simulink model "flightControlSystem"  (R2019a)
settings: Solver=ode3  StartTime=0  StopTime=TFinal  FixedStep=Ts  RelTol=1e-3  EnableMultiTasking=on
undefined symbols (not defined in the file): codertarget, controlModePosVSOrient, enableLanding, Estimator, landCommand, landingAltitude, live_time_ticks, orient_ref, pos_ref, Rec, SDTV, takeoff_flag, takeoffCommand, takeOffDuration, TFinal, Ts, x_target, y_target, z_target
libraries: simulink x5, parrotlib x3, SignalEditorBlockLib x1, sharedtransform x1, visionstatistics x1, visionconversions x1
settings Model: ExtModeTrigDuration=80  Creator=The MathWorks, Inc.  LastModifiedBy=umwan492
settings DataIOCC: LimitDataPoints=on  SaveFormat=StructureWithTime  ReturnWorkspaceOutputs=off
settings OptimizationCC: BlockReduction=off  EnhancedBackFolding=on  PassReuseOutputArgsAs=Individual arguments  MaxStackSize=64  OptimizeBlockOrder=speed  DifferentSizesBufferReuse=on  OptimizationCustomize=off
settings DebuggingCC: AlgebraicLoopMsg=none  IntegerOverflowMsg=none  ParameterPrecisionLossMsg=none  ParameterTunabilityLossMsg=error  UnconnectedInputMsg=none  UnconnectedOutputMsg=none  UnconnectedLineMsg=none  BusObjectLabelMismatch=error  PregeneratedLibrarySubsystemCodeDiagnostic=none  SFUnexpectedBacktrackingDiag=warning  SFNoUnconditionalDefaultTransitionDiag=warning  SFExecutionAtInitializationDiag=none  IntegerSaturationMsg=none  ArithmeticOperatorsInVariantConditions=warning
settings HardwareCC: ProdBitPerPointer=32  ProdBitPerSizeT=32  ProdBitPerPtrDiffT=32  ProdLargestAtomicInteger=Long  ProdWordSize=32  ProdHWDeviceType=ARM Compatible->ARM 9
settings ModelReferenceCC: ModelReferenceNumInstancesAllowed=Single  PropagateSignalLabelsOutOfModel=off
settings SFSimCC: SimUseLocalCustomCode=off  MATLABDynamicMemAlloc=off
settings RTWCC: SystemTargetFile=ert.tlc  HardwareBoard=PARROT Mambo  TLCOptions=-aInlineSetEventsForThisBaseRateFcn=TLC_FALSE -aSuppressMultiTaskScheduler=TLC_FALSE -aRateBasedStepFcn=1  TemplateMakefile=ert_default_tmf  GenerateReport=on  RTWUseLocalCustomCode=off  Toolchain=Sourcery G++ Lite GNU Toolchain for Drones  IncludeHyperlinkInReport=on  LaunchReport=on  GenerateTraceInfo=on  GenerateTraceReport=on  GenerateTraceReportSl=on  GenerateTraceReportSf=on  GenerateTraceReportEml=on
settings CodeAppCC: ForceParamTrailComments=on  IgnoreCustomStorageClasses=off  MaxIdLength=63  OperatorAnnotations=on  SimulinkDataObjDesc=on  SFDataObjDesc=on  InsertBlockDesc=on
settings ERTTargetCC: MatFileLogging=on  SupportContinuousTime=on
settings ConfigComp: CovMetricSettings=dw  CovHtmlReporting=on  CovSaveCumulativeToWorkspaceVar=on  CovSaveSingleToWorkspaceVar=on  CovExternalEMLEnable=off  CovSFcnEnable=off

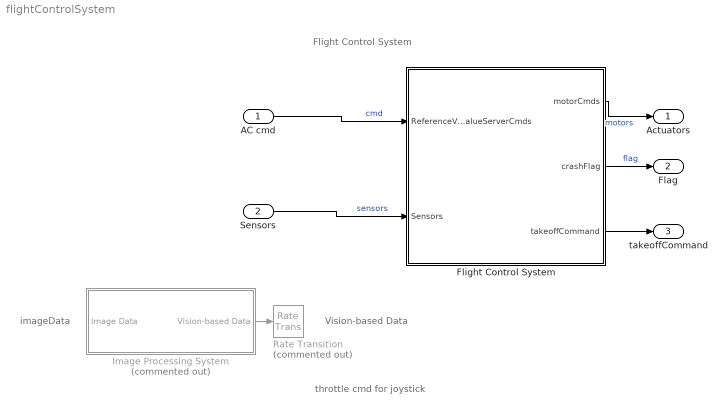
== system flightControlSystem ==
  note: throttle cmd for joystick
  note: Vision-based Data
  note: imageData
  note: Flight Control System
  AC cmd : Inport  OutDataTypeStr=Bus: CommandBus  BusOutputAsStruct=on
  Sensors : Inport  Port=2  OutDataTypeStr=Bus: SensorsBus  BusOutputAsStruct=on
  Flight Control System : Subsystem  TreatAsAtomicUnit=on
  Image Processing System : Subsystem  Tag=IP_SUB  Commented=on  InitFcn=codertarget.parrot.internal.ipSubsystemCallback(gcb);  TreatAsAtomicUnit=on  SystemSampleTime=40*Ts  RTWFcnName=ImageFunction
      settings: RTWSystemCode=Inline  RTWFcnNameOpts=User specified
  Rate Transition : RateTransition  Commented=on  Deterministic=off
  Actuators : Outport  OutDataTypeStr=single  PortDimensions=4
  Flag : Outport  Port=2  OutDataTypeStr=uint8  PortDimensions=1
  takeoffCommand : Outport  Port=3  OutDataTypeStr=boolean  PortDimensions=1
  wires:
  AC cmd/1 -> Flight Control System/1(ReferenceValueServerCmds)  "cmd"
  Flight Control System/1(motorCmds) -> Actuators/1  "motors"
  Sensors/1 -> Flight Control System/2(Sensors)  "sensors"
  Flight Control System/2(crashFlag) -> Flag/1  "flag"
  Image Processing System/1(Vision-based Data) -> Rate Transition/1
  Flight Control System/3(takeoffCommand) -> takeoffCommand/1

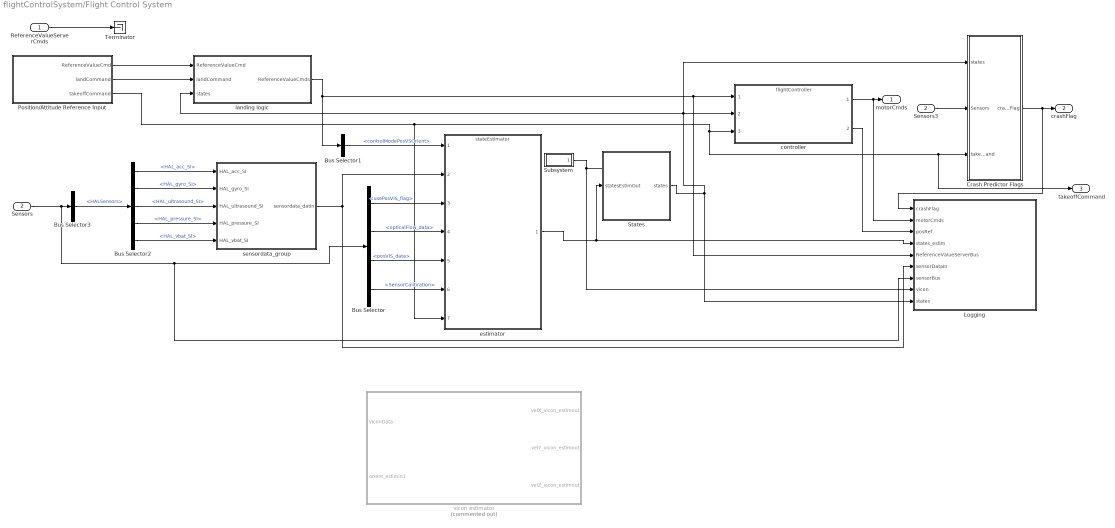
== system flightControlSystem/Flight Control System ==
  ReferenceValueServerCmds : Inport  OutDataTypeStr=Bus: CommandBus
  Sensors : Inport  Port=2  OutDataTypeStr=Bus: SensorsBus  BusOutputAsStruct=on
  Bus Selector : BusSelector  OutputSignals=VisionSensors.usePosVIS_flag,VisionSensors.opticalFlow_data,VisionSensors.posVIS_data,SensorCalibration
  Bus Selector1 : BusSelector  OutputSignals=controlModePosVSOrient
  Bus Selector2 : BusSelector  OutputSignals=HAL_acc_SI,HAL_gyro_SI,HAL_ultrasound_SI,HAL_pressure_SI,HAL_vbat_SI
  Bus Selector3 : BusSelector  OutputSignals=HALSensors
  Crash Predictor Flags : Subsystem
  Logging : Subsystem  TreatAsAtomicUnit=on
      settings: RTWFcnNameOpts=Use subsystem name
  Position/Attitude Reference Input : Subsystem
  Sensors3 : InportShadow  Port=2  OutDataTypeStr=Bus: SensorsBus  BusOutputAsStruct=on
  States : Subsystem
  Subsystem : Subsystem
  Terminator : Terminator
  controller : ModelReference  ModelNameDialog=flightController.slx  SimulationMode=Normal  ModelReferenceVersion=1.190
  estimator : ModelReference  ModelNameDialog=stateEstimator.slx  SimulationMode=Normal  ModelReferenceVersion=1.78
  landing logic : Subsystem
  sensordata_group : Subsystem
  vicon estimator : Subsystem  Commented=on
  motorCmds : Outport
  crashFlag : Outport  Port=2
  takeoffCommand : Outport  Port=3  OutDataTypeStr=boolean
  wires:
  Bus Selector2/1 -> sensordata_group/1(HAL_acc_SI)  "<HAL_acc_SI>"
  Bus Selector2/2 -> sensordata_group/2(HAL_gyro_SI)  "<HAL_gyro_SI>"
  Bus Selector2/4 -> sensordata_group/4(HAL_pressure_SI)  "<HAL_pressure_SI>"
  Bus Selector2/3 -> sensordata_group/3(HAL_ultrasound_SI)  "<HAL_ultrasound_SI>"
  estimator/1 -> States/1(statesEstimOut), Logging/4(states_estim)
  controller/2 -> Logging/3(posRef)
  landing logic/1(ReferenceValueCmds) -> Logging/5(ReferenceValueServerBus), controller/1, Bus Selector1/1
  controller/1 -> motorCmds/1, Logging/2(motorCmds)
  sensordata_group/1(sensordata_datin) -> Logging/6(sensorDataIn), estimator/2
  Bus Selector2/5 -> sensordata_group/5(HAL_vbat_SI)  "<HAL_vbat_SI>"
  Crash Predictor Flags/1(crashFlag) -> Logging/1(crashFlag), crashFlag/1
  Sensors/1 -> Logging/7(sensorBus), Bus Selector/1, Bus Selector3/1
  Bus Selector3/1 -> Bus Selector2/1  "<HALSensors>"
  Bus Selector/1 -> estimator/3  "<usePosVIS_flag>"
  Bus Selector/2 -> estimator/4  "<opticalFlow_data>"
  Bus Selector/3 -> estimator/5  "<posVIS_data>"
  Bus Selector/4 -> estimator/6  "<SensorCalibration>"
  Bus Selector1/1 -> estimator/1  "<controlModePosVSOrient>"
  ReferenceValueServerCmds/1 -> Terminator/1
  Position/Attitude Reference Input/1(ReferenceValueCmd) -> landing logic/1(ReferenceValueCmd)
  Sensors3/1 -> Crash Predictor Flags/2(Sensors)
  States/1(states) -> controller/2, landing logic/3(states), Crash Predictor Flags/1(states), Logging/9(states)
  Subsystem/1(viconData) -> Logging/8(vicon)
  Position/Attitude Reference Input/2(landCommand) -> landing logic/2(landCommand)
  Position/Attitude Reference Input/3(takeoffCommand) -> estimator/7, controller/3, takeoffCommand/1, Crash Predictor Flags/3(takeoffCommand)

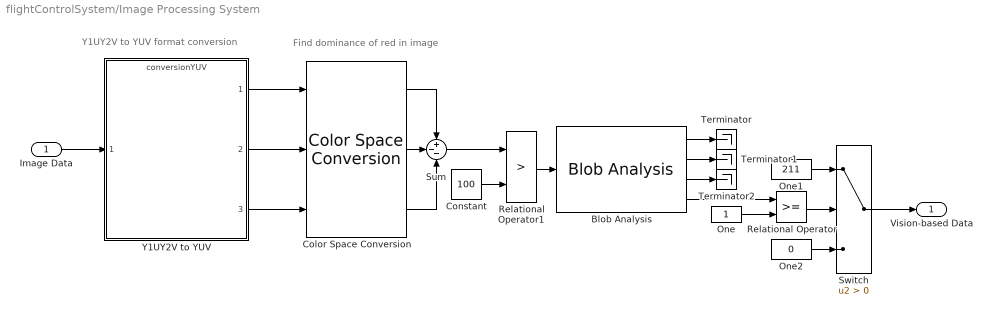
== system flightControlSystem/Image Processing System ==
  note: Find dominance of red in image
  note: Y1UY2V to YUV format conversion
  Image Data : Inport
  Blob Analysis : visionstatistics/Blob Analysis  Tag=vipblks_row_conv  area=on  centroid=on  bBox=on  majorAxis=off  minorAxis=off  angle=off  eccentricity=off  equivDiameterSq=off  extent=off  perimeter=off  outDT=single  conn=8  isLabel=off  maxBlobs=50  warnIfNumBlobsExceeded=on  isCount=on  useMinArea=off  minArea=0  useMaxArea=off  maxArea=intmax('uint32')  excludeBorderBlob=off  isOutVarDim=off  isFill=on  fillValues=-1  roundingMode=Floor  overflowMode=off  prodOutputMode=Binary point scaling  prodOutputWordLength=32  prodOutputFracLength=16  prodOutputSlope=2^-16  accumMode=Binary point scaling  accumWordLength=32  accumFracLength=0  accumSlope=2^0  outputMode=Binary point scaling  outputWordLength=32  outputFracLength=16  outputSlope=2^-16  memorySlope=2^-16  firstCoeffMode=Binary point scaling  firstCoeffWordLength=16  firstCoeffFracLength=14  firstCoeffSlope=2^-14  secondCoeffMode=Binary point scaling  secondCoeffWordLength=32  secondCoeffFracLength=16  secondCoeffSlope=2^-16
      settings: SourceProductName=Computer Vision Toolbox
  Color Space Conversion : visionconversions/Color Space  Conversion  conversion=Obsolete  conversionActive=Y'CbCr to R'G'B'  wp_str=D65  rec=Rec. 601 (SDTV)  sys=1125/60/2:1  imagePorts=Separate color signals
  Constant : Constant  Value=100  OutDataTypeStr=uint8
  One : Constant  OutDataTypeStr=Inherit: Inherit via back propagation
  One1 : Constant  Value=211  OutDataTypeStr=Inherit: Inherit via back propagation
  One2 : Constant  Value=0  OutDataTypeStr=Inherit: Inherit via back propagation
  Relational Operator : RelationalOperator  OutDataTypeStr=boolean  RndMeth=Simplest
  Relational Operator1 : RelationalOperator  Operator=>  OutDataTypeStr=boolean  RndMeth=Simplest
  Sum : Sum  Inputs=+--  SaturateOnIntegerOverflow=on
  Switch : Switch  Criteria=u2 > Threshold
  Terminator : Terminator
  Terminator1 : Terminator
  Terminator2 : Terminator
  Y1UY2V to YUV : ModelReference  ModelNameDialog=conversionYUV.slx  SimulationMode=Normal  ModelReferenceVersion=1.145
  Vision-based Data : Outport
  wires:
  One/1 -> Relational Operator/2
  Blob Analysis/4 -> Relational Operator/1
  Relational Operator1/1 -> Blob Analysis/1
  Color Space Conversion/1 -> Sum/1
  Color Space Conversion/2 -> Sum/2
  Color Space Conversion/3 -> Sum/3
  Sum/1 -> Relational Operator1/1
  Constant/1 -> Relational Operator1/2
  Blob Analysis/1 -> Terminator/1
  Blob Analysis/2 -> Terminator1/1
  Blob Analysis/3 -> Terminator2/1
  Relational Operator/1 -> Switch/2
  Switch/1 -> Vision-based Data/1
  One1/1 -> Switch/1
  One2/1 -> Switch/3
  Image Data/1 -> Y1UY2V to YUV/1
  Y1UY2V to YUV/1 -> Color Space Conversion/1
  Y1UY2V to YUV/2 -> Color Space Conversion/2
  Y1UY2V to YUV/3 -> Color Space Conversion/3

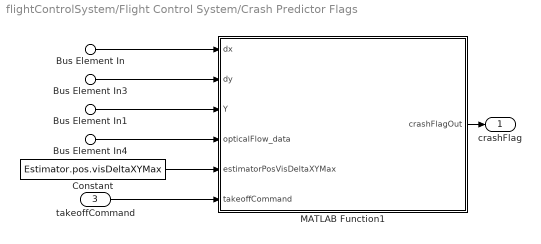
== system flightControlSystem/Flight Control System/Crash Predictor Flags ==
  Bus Element In1 : Inport  PortName=states  Element=Y
  Bus Element In : Inport  PortName=states  Element=dx
  Bus Element In3 : Inport  PortName=states  Element=dy
  Bus Element In4 : Inport  Port=2  PortName=Sensors  Element=VisionSensors.opticalFlow_data
  takeoffCommand : Inport  Port=3
  Constant : Constant  Value=Estimator.pos.visDeltaXYMax
  MATLAB Function1 : MATLAB Function  TreatAsAtomicUnit=on
  crashFlag : Outport
  wires:
  Bus Element In4/1 -> MATLAB Function1/4(opticalFlow_data)
  MATLAB Function1/1(crashFlagOut) -> crashFlag/1
  Bus Element In3/1 -> MATLAB Function1/2(dy)
  Constant/1 -> MATLAB Function1/5(estimatorPosVisDeltaXYMax)
  Bus Element In/1 -> MATLAB Function1/1(dx)
  takeoffCommand/1 -> MATLAB Function1/6(takeoffCommand)
  Bus Element In1/1 -> MATLAB Function1/3(Y)

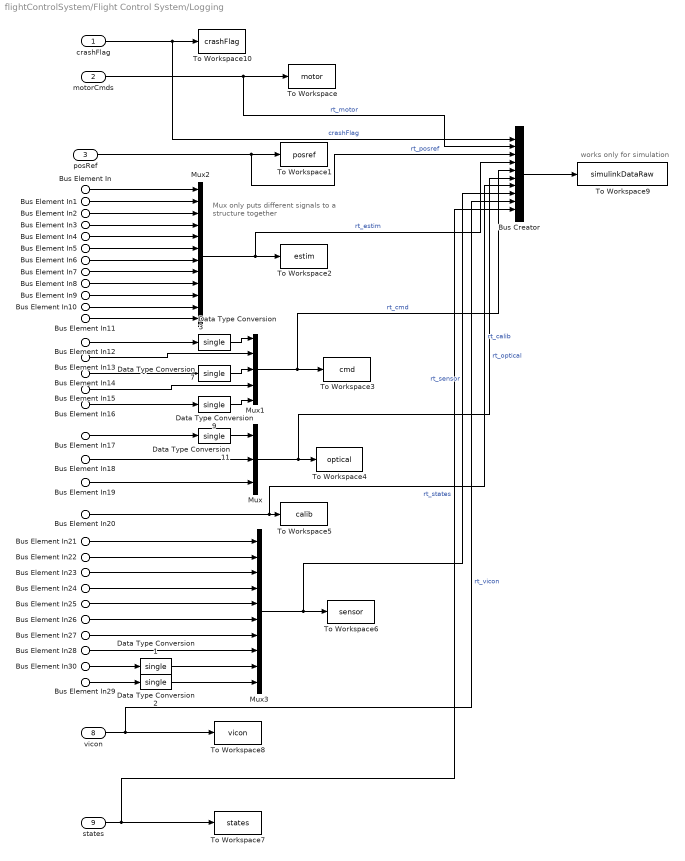
== system flightControlSystem/Flight Control System/Logging ==
  note: works only for simulation
  note: Mux only puts different signals to a structure together
  crashFlag : Inport
  motorCmds : Inport  Port=2
  posRef : Inport  Port=3
  Bus Element In : Inport  Port=4  PortName=states_estim  Element=X
  Bus Element In1 : Inport  Port=4  PortName=states_estim  Element=Y
  Bus Element In2 : Inport  Port=4  PortName=states_estim  Element=Z
  Bus Element In3 : Inport  Port=4  PortName=states_estim  Element=yaw
  Bus Element In6 : Inport  Port=4  PortName=states_estim  Element=dx
  Bus Element In5 : Inport  Port=4  PortName=states_estim  Element=roll
  Bus Element In4 : Inport  Port=4  PortName=states_estim  Element=pitch
  Bus Element In7 : Inport  Port=4  PortName=states_estim  Element=dy
  Bus Element In8 : Inport  Port=4  PortName=states_estim  Element=dz
  Bus Element In9 : Inport  Port=4  PortName=states_estim  Element=p
  Bus Element In10 : Inport  Port=4  PortName=states_estim  Element=q
  Bus Element In11 : Inport  Port=4  PortName=states_estim  Element=r
  Bus Element In12 : Inport  Port=5  PortName=ReferenceValueServerBus  Element=controlModePosVSOrient
  Bus Element In13 : Inport  Port=5  PortName=ReferenceValueServerBus  Element=pos_ref
  Bus Element In14 : Inport  Port=5  PortName=ReferenceValueServerBus  Element=takeoff_flag
  Bus Element In15 : Inport  Port=5  PortName=ReferenceValueServerBus  Element=orient_ref
  Bus Element In16 : Inport  Port=5  PortName=ReferenceValueServerBus  Element=live_time_ticks
  Bus Element In21 : Inport  Port=6  PortName=sensorDataIn  Element=ddx
  Bus Element In22 : Inport  Port=6  PortName=sensorDataIn  Element=ddy
  Bus Element In23 : Inport  Port=6  PortName=sensorDataIn  Element=ddz
  Bus Element In24 : Inport  Port=6  PortName=sensorDataIn  Element=p
  Bus Element In25 : Inport  Port=6  PortName=sensorDataIn  Element=q
  Bus Element In26 : Inport  Port=6  PortName=sensorDataIn  Element=r
  Bus Element In27 : Inport  Port=6  PortName=sensorDataIn  Element=altitude_sonar
  Bus Element In28 : Inport  Port=6  PortName=sensorDataIn  Element=prs
  Bus Element In29 : Inport  Port=6  PortName=sensorDataIn  Element=vbat_percentage
  Bus Element In30 : Inport  Port=6  PortName=sensorDataIn  Element=vbat_V
  Bus Element In17 : Inport  Port=7  PortName=sensorBus  Element=VisionSensors.usePosVIS_flag
  Bus Element In18 : Inport  Port=7  PortName=sensorBus  Element=VisionSensors.opticalFlow_data
  Bus Element In19 : Inport  Port=7  PortName=sensorBus  Element=VisionSensors.posVIS_data
  Bus Element In20 : Inport  Port=7  PortName=sensorBus  Element=SensorCalibration
  vicon : Inport  Port=8  OutDataTypeStr=Bus: viconData
  states : Inport  Port=9  OutDataTypeStr=Bus: statesBB
  Bus Creator : BusCreator  Inputs=10
  Data Type Conversion{1..3,7,9,11} (6 alike) : DataTypeConversion  OutDataTypeStr=single
  Mux : Mux  Inputs=3
  Mux1 : Mux  Inputs=5
  Mux2 : Mux  Inputs=12
  Mux3 : Mux  Inputs=10
  To Workspace : ToWorkspace  VariableName=motor  SaveFormat=Structure With Time  SampleTime=-1
  To Workspace1 : ToWorkspace  VariableName=posref  SaveFormat=Structure With Time  SampleTime=-1
  To Workspace10 : ToWorkspace  VariableName=crashFlag  SaveFormat=Structure With Time  SampleTime=-1
  To Workspace2 : ToWorkspace  VariableName=estim  SaveFormat=Structure With Time  SampleTime=-1
  To Workspace3 : ToWorkspace  VariableName=cmd  SaveFormat=Structure With Time  SampleTime=-1
  To Workspace4 : ToWorkspace  VariableName=optical  SaveFormat=Structure With Time  SampleTime=-1
  To Workspace5 : ToWorkspace  VariableName=calib  SaveFormat=Structure With Time  SampleTime=-1
      settings: Decimation=100
  To Workspace6 : ToWorkspace  VariableName=sensor  SaveFormat=Structure With Time  SampleTime=-1
  To Workspace7 : ToWorkspace  VariableName=states  SaveFormat=Structure With Time  SampleTime=-1
  To Workspace8 : ToWorkspace  VariableName=vicon  SaveFormat=Structure With Time  SampleTime=-1
  To Workspace9 : ToWorkspace  VariableName=simulinkDataRaw  SaveFormat=Timeseries  SampleTime=-1
  wires:
  Bus Element In12/1 -> Data Type Conversion3/1
  Bus Element In14/1 -> Data Type Conversion7/1
  Bus Element In16/1 -> Data Type Conversion9/1
  Bus Element In17/1 -> Data Type Conversion11/1
  Bus Element In20/1 -> Bus Creator/7, To Workspace5/1  "rt_calib"
  Mux/1 -> Bus Creator/6, To Workspace4/1  "rt_optical"
  Mux2/1 -> Bus Creator/4, To Workspace2/1  "rt_estim"
  motorCmds/1 -> Bus Creator/2, To Workspace/1  "rt_motor"
  Mux1/1 -> Bus Creator/5, To Workspace3/1  "rt_cmd"
  Bus Element In3/1 -> Mux2/4
  Bus Element In5/1 -> Mux2/6
  Bus Element In4/1 -> Mux2/5
  Bus Element In8/1 -> Mux2/9
  Bus Element In6/1 -> Mux2/7
  Bus Element In7/1 -> Mux2/8
  Bus Element In9/1 -> Mux2/10
  Bus Element In11/1 -> Mux2/12
  Bus Element In1/1 -> Mux2/2
  Bus Element In10/1 -> Mux2/11
  Bus Element In2/1 -> Mux2/3
  Bus Element In/1 -> Mux2/1
  Data Type Conversion3/1 -> Mux1/1
  Bus Element In13/1 -> Mux1/2
  Data Type Conversion7/1 -> Mux1/3
  Bus Element In15/1 -> Mux1/4
  Data Type Conversion9/1 -> Mux1/5
  Bus Element In19/1 -> Mux/3
  Bus Element In18/1 -> Mux/2
  Data Type Conversion11/1 -> Mux/1
  posRef/1 -> Bus Creator/3, To Workspace1/1  "rt_posref"
  Bus Element In21/1 -> Mux3/1
  Bus Element In22/1 -> Mux3/2
  Bus Element In23/1 -> Mux3/3
  Bus Element In24/1 -> Mux3/4
  Bus Element In25/1 -> Mux3/5
  Bus Element In26/1 -> Mux3/6
  Bus Element In27/1 -> Mux3/7
  Bus Element In28/1 -> Mux3/8
  Bus Element In30/1 -> Data Type Conversion1/1
  Bus Element In29/1 -> Data Type Conversion2/1
  Mux3/1 -> Bus Creator/8, To Workspace6/1  "rt_sensor"
  Data Type Conversion1/1 -> Mux3/9
  Data Type Conversion2/1 -> Mux3/10
  states/1 -> Bus Creator/10, To Workspace7/1  "rt_states"
  vicon/1 -> Bus Creator/9, To Workspace8/1  "rt_vicon"
  Bus Creator/1 -> To Workspace9/1
  crashFlag/1 -> Bus Creator/1, To Workspace10/1  "crashFlag"

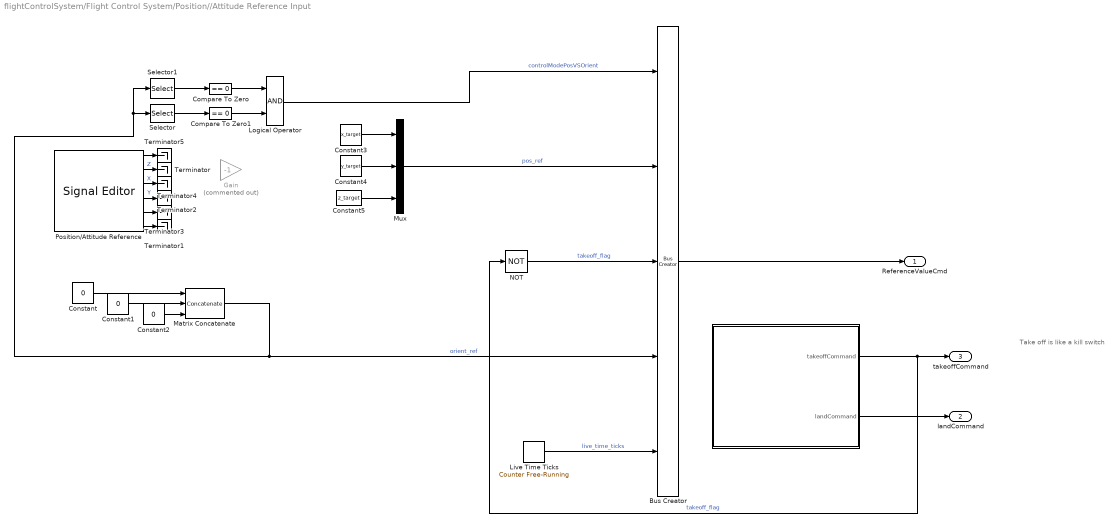
== system flightControlSystem/Flight Control System/Position//Attitude Reference Input ==
  note: Take off is like a kill switch
  " " : Subsystem  Variant=on  VariantControl=Variant1
  Bus Creator : BusCreator  Inputs=controlModePosVSOrient,pos_ref,takeoff_flag,orient_ref,live_time_ticks  OutDataTypeStr=Bus: CommandBus  NonVirtualBus=on
  Compare To Zero : simulink/Logic and Bit Operations/Compare To Zero  relop===  OutDataTypeStr=boolean
  Compare To Zero1 : simulink/Logic and Bit Operations/Compare To Zero  relop===  OutDataTypeStr=boolean
  Constant : Constant  Value=0  OutDataTypeStr=single  SampleTime=Ts
  Constant1 : Constant  Value=0  OutDataTypeStr=single  SampleTime=Ts
  Constant2 : Constant  Value=0  OutDataTypeStr=single  SampleTime=Ts
  Constant3 : Constant  Value=x_target  OutDataTypeStr=single  SampleTime=Ts
  Constant4 : Constant  Value=y_target  OutDataTypeStr=single  SampleTime=Ts
  Constant5 : Constant  Value=z_target  OutDataTypeStr=single  SampleTime=Ts
  Gain : Gain  Commented=on  Gain=-1
  Live Time Ticks : simulink/Sources/Counter Free-Running  NumBits=32  tsamp=Ts
  Logical Operator : Logic  AllPortsSameDT=off  OutDataTypeStr=boolean
  Matrix Concatenate : Concatenate  NumInputs=3  Mode=Multidimensional array  ConcatenateDimension=2
  Mux : Mux  Inputs=3
  NOT : Logic  Operator=NOT  IconShape=distinctive  AllPortsSameDT=off  OutDataTypeStr=boolean
  Position/Attitude Reference : SignalEditorBlockLib/Signal Editor  FileName=positionAttitudeRef.mat  ActiveScenario=Amin_Hover  ActiveSignal=Signal  IsBus=off  OutputBusObjectStr=Bus: BusObject  SampleTime=Ts  ZeroCross=off  OutputAfterFinalValue=Setting to zero  Unit=inherit  PreserveSignalName=on
      settings: SourceProductName=Simulink
  Selector : Selector  InputPortWidth=3  IndexOptions=Index vector (dialog)  Indices=2  OutputSizes=1
  Selector1 : Selector  InputPortWidth=3  IndexOptions=Index vector (dialog)  Indices=3  OutputSizes=1
  Terminator{,1..5} (6 alike) : Terminator
  ReferenceValueCmd : Outport
  landCommand : Outport  Port=2
  takeoffCommand : Outport  Port=3
  wires:
  Logical Operator/1 -> Bus Creator/1  "controlModePosVSOrient"
  Selector/1 -> Compare To Zero1/1
  Live Time Ticks/1 -> Bus Creator/5  "live_time_ticks"
  Compare To Zero1/1 -> Logical Operator/2
  Selector1/1 -> Compare To Zero/1
  Compare To Zero/1 -> Logical Operator/1
  Matrix Concatenate/1 -> Selector1/1, Selector/1, Bus Creator/4  "orient_ref"
  Constant/1 -> Matrix Concatenate/1
  Constant1/1 -> Matrix Concatenate/2
  Constant2/1 -> Matrix Concatenate/3
  Constant3/1 -> Mux/1
  Constant4/1 -> Mux/2
  Position/Attitude Reference/2 -> Terminator/1  "Z"
  Position/Attitude Reference/4 -> Terminator2/1  "Y"
  Position/Attitude Reference/5 -> Terminator3/1
  Position/Attitude Reference/6 -> Terminator1/1
  Position/Attitude Reference/3 -> Terminator4/1  "X"
  Position/Attitude Reference/1 -> Terminator5/1
  Constant5/1 -> Mux/3
  Mux/1 -> Bus Creator/2  "pos_ref"
  Bus Creator/1 -> ReferenceValueCmd/1
  " "/1(takeoffCommand) -> NOT/1, takeoffCommand/1  "takeoff_flag"
  " "/2(landCommand) -> landCommand/1
  NOT/1 -> Bus Creator/3  "takeoff_flag"

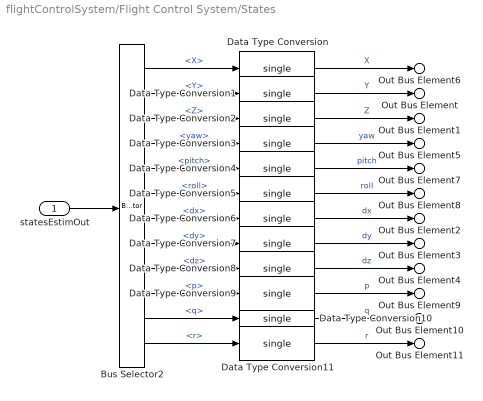
== system flightControlSystem/Flight Control System/States ==
  statesEstimOut : Inport  OutDataTypeStr=Bus: statesEstim_t
  Bus Selector2 : BusSelector  OutputSignals=X,Y,Z,yaw,pitch,roll,dx,dy,dz,p,q,r
  Data Type Conversion{,1..11} (12 alike) : DataTypeConversion  OutDataTypeStr=single
  Out Bus Element6 : Outport  PortName=states  Element=X
  Out Bus Element : Outport  PortName=states  Element=Y
  Out Bus Element1 : Outport  PortName=states  Element=Z
  Out Bus Element5 : Outport  PortName=states  Element=yaw
  Out Bus Element7 : Outport  PortName=states  Element=pitch
  Out Bus Element8 : Outport  PortName=states  Element=roll
  Out Bus Element2 : Outport  PortName=states  Element=dx
  Out Bus Element3 : Outport  PortName=states  Element=dy
  Out Bus Element4 : Outport  PortName=states  Element=dz
  Out Bus Element9 : Outport  PortName=states  Element=p
  Out Bus Element10 : Outport  PortName=states  Element=q
  Out Bus Element11 : Outport  PortName=states  Element=r
  wires:
  statesEstimOut/1 -> Bus Selector2/1
  Bus Selector2/1 -> Data Type Conversion/1  "<X>"
  Bus Selector2/2 -> Data Type Conversion1/1  "<Y>"
  Bus Selector2/3 -> Data Type Conversion2/1  "<Z>"
  Bus Selector2/4 -> Data Type Conversion3/1  "<yaw>"
  Bus Selector2/5 -> Data Type Conversion4/1  "<pitch>"
  Bus Selector2/6 -> Data Type Conversion5/1  "<roll>"
  Bus Selector2/7 -> Data Type Conversion6/1  "<dx>"
  Bus Selector2/8 -> Data Type Conversion7/1  "<dy>"
  Bus Selector2/9 -> Data Type Conversion8/1  "<dz>"
  Bus Selector2/10 -> Data Type Conversion9/1  "<p>"
  Bus Selector2/11 -> Data Type Conversion10/1  "<q>"
  Bus Selector2/12 -> Data Type Conversion11/1  "<r>"
  Data Type Conversion/1 -> Out Bus Element6/1  "X"
  Data Type Conversion1/1 -> Out Bus Element/1  "Y"
  Data Type Conversion2/1 -> Out Bus Element1/1  "Z"
  Data Type Conversion3/1 -> Out Bus Element5/1  "yaw"
  Data Type Conversion4/1 -> Out Bus Element7/1  "pitch"
  Data Type Conversion5/1 -> Out Bus Element8/1  "roll"
  Data Type Conversion6/1 -> Out Bus Element2/1  "dx"
  Data Type Conversion7/1 -> Out Bus Element3/1  "dy"
  Data Type Conversion8/1 -> Out Bus Element4/1  "dz"
  Data Type Conversion9/1 -> Out Bus Element9/1  "p"
  Data Type Conversion10/1 -> Out Bus Element10/1  "q"
  Data Type Conversion11/1 -> Out Bus Element11/1  "r"

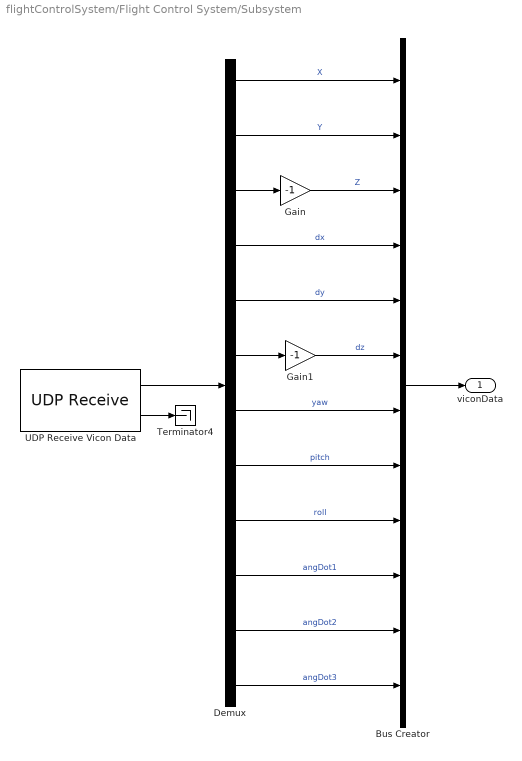
== system flightControlSystem/Flight Control System/Subsystem ==
  Bus Creator : BusCreator  Inputs=12  OutDataTypeStr=Bus: viconData
      settings: InheritFromInputs=off
  Demux : Demux  Outputs=12
  Gain : Gain  Gain=-1
  Gain1 : Gain  Gain=-1
  Terminator4 : Terminator
  UDP Receive Vicon Data : parrotlib/UDP Receive  localURL='0.0.0.0'  localPort=25000  remoteURL='0.0.0.0'  remotePort=-1  recvBufferSize=8192  signalDatatype=single  dims=12  isVarSize=off  showBlockingTime=off  blockingTime=0  sampletime=0.005  blockPlatform=LINUX
      settings: SourceProductName=Simulink Support Package for PARROT Minidrones  SourceProductBaseCode=MINIDRONES
  viconData : Outport  OutDataTypeStr=Bus: viconData
  wires:
  Demux/7 -> Bus Creator/7  "yaw"
  Demux/1 -> Bus Creator/1  "X"
  Gain/1 -> Bus Creator/3  "Z"
  Demux/10 -> Bus Creator/10  "angDot1"
  UDP Receive Vicon Data/2 -> Terminator4/1
  Demux/12 -> Bus Creator/12  "angDot3"
  Demux/5 -> Bus Creator/5  "dy"
  UDP Receive Vicon Data/1 -> Demux/1
  Demux/11 -> Bus Creator/11  "angDot2"
  Demux/2 -> Bus Creator/2  "Y"
  Gain1/1 -> Bus Creator/6  "dz"
  Demux/4 -> Bus Creator/4  "dx"
  Demux/9 -> Bus Creator/9  "roll"
  Demux/6 -> Gain1/1
  Demux/3 -> Gain/1
  Demux/8 -> Bus Creator/8  "pitch"
  Bus Creator/1 -> viconData/1

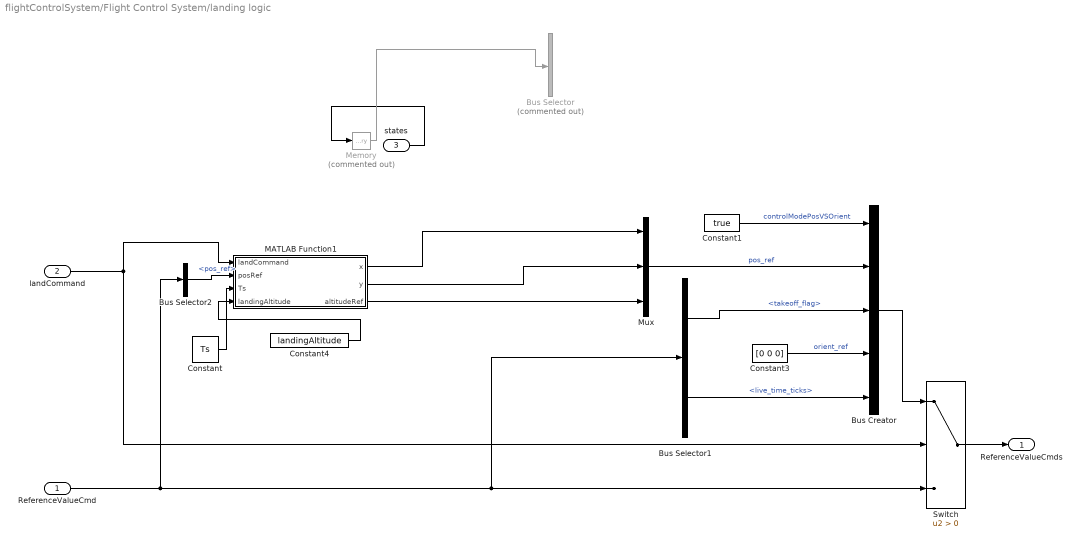
== system flightControlSystem/Flight Control System/landing logic ==
  ReferenceValueCmd : Inport
  landCommand : Inport  Port=2
  states : Inport  Port=3  OutDataTypeStr=Bus: statesBB
  Bus Creator : BusCreator  Inputs=5  OutDataTypeStr=Bus: CommandBus  NonVirtualBus=on
  Bus Selector : BusSelector  Commented=on  OutputSignals=X,Y
  Bus Selector1 : BusSelector  OutputSignals=takeoff_flag,live_time_ticks
  Bus Selector2 : BusSelector  OutputSignals=pos_ref
  Constant : Constant  Value=Ts
  Constant1 : Constant  Value=true  OutDataTypeStr=boolean
  Constant3 : Constant  Value=[0 0 0]  OutDataTypeStr=single
  Constant4 : Constant  Value=landingAltitude  OutDataTypeStr=single  SampleTime=Ts
  MATLAB Function1 : MATLAB Function  TreatAsAtomicUnit=on
  Memory : Memory  Commented=on  InheritSampleTime=on
  Mux : Mux  Inputs=3
  Switch : Switch  Criteria=u2 > Threshold
  ReferenceValueCmds : Outport  OutDataTypeStr=Bus: CommandBus
  wires:
  Switch/1 -> ReferenceValueCmds/1
  landCommand/1 -> Switch/2, MATLAB Function1/1(landCommand)
  Mux/1 -> Bus Creator/2  "pos_ref"
  Constant1/1 -> Bus Creator/1  "controlModePosVSOrient"
  Bus Selector1/1 -> Bus Creator/3  "<takeoff_flag>"
  states/1 -> Memory/1
  Bus Selector1/2 -> Bus Creator/5  "<live_time_ticks>"
  Constant3/1 -> Bus Creator/4  "orient_ref"
  Bus Creator/1 -> Switch/1
  ReferenceValueCmd/1 -> Bus Selector2/1, Bus Selector1/1, Switch/3
  Memory/1 -> Bus Selector/1
  Bus Selector2/1 -> MATLAB Function1/2(posRef)  "<pos_ref>"
  Constant/1 -> MATLAB Function1/3(Ts)
  Constant4/1 -> MATLAB Function1/4(landingAltitude)
  MATLAB Function1/3(altitudeRef) -> Mux/3
  MATLAB Function1/1(x) -> Mux/1
  MATLAB Function1/2(y) -> Mux/2

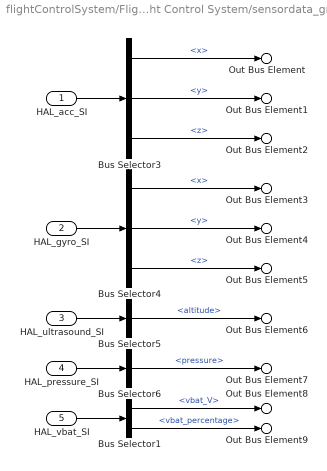
== system flightControlSystem/Flight Control System/sensordata_group ==
  HAL_acc_SI : Inport  OutDataTypeStr=Bus: HAL_acc_SI_t
  HAL_gyro_SI : Inport  Port=2  OutDataTypeStr=Bus: HAL_gyro_SI_t
  HAL_ultrasound_SI : Inport  Port=3  OutDataTypeStr=Bus: HAL_ultrasound_SI_t
  HAL_pressure_SI : Inport  Port=4  OutDataTypeStr=Bus: HAL_pressure_SI_t
  HAL_vbat_SI : Inport  Port=5  OutDataTypeStr=Bus: HAL_vbat_SI_t
  Bus Selector1 : BusSelector  OutputSignals=vbat_V,vbat_percentage
  Bus Selector3 : BusSelector  OutputSignals=x,y,z
  Bus Selector4 : BusSelector  OutputSignals=x,y,z
  Bus Selector5 : BusSelector  OutputSignals=altitude
  Bus Selector6 : BusSelector  OutputSignals=pressure
  Out Bus Element : Outport  PortName=sensordata_datin  Element=ddx
  Out Bus Element1 : Outport  PortName=sensordata_datin  Element=ddy
  Out Bus Element2 : Outport  PortName=sensordata_datin  Element=ddz
  Out Bus Element3 : Outport  PortName=sensordata_datin  Element=p
  Out Bus Element4 : Outport  PortName=sensordata_datin  Element=q
  Out Bus Element5 : Outport  PortName=sensordata_datin  Element=r
  Out Bus Element6 : Outport  PortName=sensordata_datin  Element=altitude_sonar
  Out Bus Element7 : Outport  PortName=sensordata_datin  Element=prs
  Out Bus Element8 : Outport  PortName=sensordata_datin  Element=vbat_V
  Out Bus Element9 : Outport  PortName=sensordata_datin  Element=vbat_percentage
  wires:
  HAL_gyro_SI/1 -> Bus Selector4/1
  HAL_acc_SI/1 -> Bus Selector3/1
  HAL_pressure_SI/1 -> Bus Selector6/1
  HAL_ultrasound_SI/1 -> Bus Selector5/1
  Bus Selector4/1 -> Out Bus Element3/1  "<x>"
  Bus Selector3/3 -> Out Bus Element2/1  "<z>"
  Bus Selector4/3 -> Out Bus Element5/1  "<z>"
  Bus Selector5/1 -> Out Bus Element6/1  "<altitude>"
  Bus Selector6/1 -> Out Bus Element7/1  "<pressure>"
  Bus Selector4/2 -> Out Bus Element4/1  "<y>"
  Bus Selector3/1 -> Out Bus Element/1  "<x>"
  Bus Selector3/2 -> Out Bus Element1/1  "<y>"
  Bus Selector1/1 -> Out Bus Element8/1  "<vbat_V>"
  HAL_vbat_SI/1 -> Bus Selector1/1
  Bus Selector1/2 -> Out Bus Element9/1  "<vbat_percentage>"

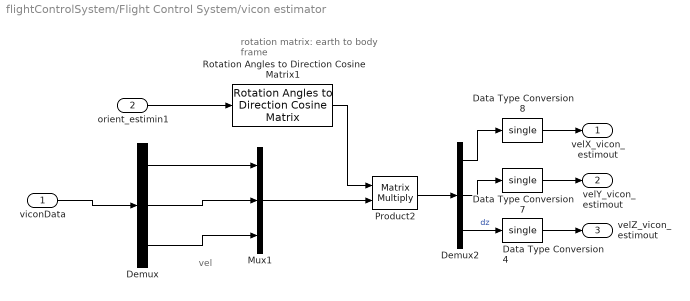
== system flightControlSystem/Flight Control System/vicon estimator ==
  note: rotation matrix:
      | earth to body frame
  note: vel
  viconData : Inport
  orient_estimin1 : Inport  Port=2
  Data Type Conversion4 : DataTypeConversion  OutDataTypeStr=single  SaturateOnIntegerOverflow=on
  Data Type Conversion7 : DataTypeConversion  OutDataTypeStr=single  SaturateOnIntegerOverflow=on
  Data Type Conversion8 : DataTypeConversion  OutDataTypeStr=single  SaturateOnIntegerOverflow=on
  Demux : Demux  Outputs=3  BusSelectionMode=on
  Demux2 : Demux  Outputs=3
  Mux1 : Mux  Inputs=3
  Product2 : Product  Multiplication=Matrix(*)
  Rotation Angles to Direction Cosine Matrix1 : sharedtransform/Rotation Angles to Direction Cosine Matrix  rotationOrder=ZYX  aMode=aMode
      settings: SourceProductBaseCode=AE
  velX_vicon_estimout : Outport
  velY_vicon_estimout : Outport  Port=2
  velZ_vicon_estimout : Outport  Port=3
  wires:
  Demux2/2 -> Data Type Conversion7/1
  orient_estimin1/1 -> Rotation Angles to Direction Cosine Matrix1/1
  Data Type Conversion8/1 -> velX_vicon_estimout/1
  Data Type Conversion7/1 -> velY_vicon_estimout/1
  Product2/1 -> Demux2/1
  Demux2/3 -> Data Type Conversion4/1  "dz"
  Mux1/1 -> Product2/2
  Demux2/1 -> Data Type Conversion8/1
  Rotation Angles to Direction Cosine Matrix1/1 -> Product2/1
  Data Type Conversion4/1 -> velZ_vicon_estimout/1
  viconData/1 -> Demux/1
  Demux/1 -> Mux1/1
  Demux/2 -> Mux1/2
  Demux/3 -> Mux1/3

== system flightControlSystem/Flight Control System/Position//Attitude Reference Input/  ==
  note: One block becomes active based on VSS_RunMode and VSS_ControlMode
  keyboard Commands : Subsystem  VariantControl=VSS_ControlMode==1 && VSS_RunMode==1
  simulation keyboard : Subsystem  VariantControl=VSS_ControlMode==1 && VSS_RunMode==0
  time based : Subsystem  VariantControl=VSS_ControlMode==0
  takeoffCommand : Outport
  landCommand : Outport  Port=2

== system flightControlSystem/Flight Control System/Position//Attitude Reference Input/ /keyboard Commands ==
  note: if joystick use throttle for altitude input
  Constant : Constant  Value=enableLanding
  Keyboard Read1 : parrotlib/Keyboard Read  Commented=on  SampleTime_=0.005
      settings: SourceProductName=Simulink Support Package for PARROT Minidrones  SourceProductBaseCode=MINIDRONES
  MATLAB Function : MATLAB Function  TreatAsAtomicUnit=on
  Terminator : Terminator
  UDP Receive : parrotlib/UDP Receive  localURL='0.0.0.0'  localPort=26061  remoteURL='0.0.0.0'  remotePort=-1  recvBufferSize=8192  signalDatatype=uint8  dims=1  isVarSize=off  showBlockingTime=off  blockingTime=0  sampletime=0.005  blockPlatform=LINUX
      settings: SourceProductName=Simulink Support Package for PARROT Minidrones  SourceProductBaseCode=MINIDRONES
  takeoffCommand : Outport
  landCommand : Outport  Port=2
  wires:
  UDP Receive/1 -> MATLAB Function/1(keyboardRead)  "KeyboardRead"
  UDP Receive/2 -> Terminator/1
  Constant/1 -> MATLAB Function/2(enableLanding)
  MATLAB Function/1(landCommand) -> landCommand/1
  MATLAB Function/2(takeoffCommand) -> takeoffCommand/1

== system flightControlSystem/Flight Control System/Position//Attitude Reference Input/ /simulation keyboard ==
  Constant : Constant  Value=takeoffCommand
  Constant1 : Constant  Value=landCommand
  takeoffCommand : Outport
  landCommand : Outport  Port=2
  wires:
  Constant1/1 -> landCommand/1  "land"
  Constant/1 -> takeoffCommand/1  "takeoff"

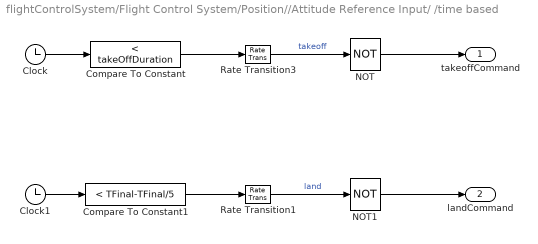
== system flightControlSystem/Flight Control System/Position//Attitude Reference Input/ /time based ==
  Clock : Clock
  Clock1 : Clock
  Compare To Constant : simulink/Logic and Bit Operations/Compare To Constant  relop=<  const=takeOffDuration  OutDataTypeStr=boolean
  Compare To Constant1 : simulink/Logic and Bit Operations/Compare To Constant  relop=<  const=TFinal-TFinal/5  OutDataTypeStr=boolean
  NOT : Logic  Operator=NOT  IconShape=distinctive  AllPortsSameDT=off  OutDataTypeStr=boolean
  NOT1 : Logic  Operator=NOT  IconShape=distinctive  AllPortsSameDT=off  OutDataTypeStr=boolean
  Rate Transition1 : RateTransition  OutPortSampleTime=Ts
  Rate Transition3 : RateTransition  OutPortSampleTime=Ts
  takeoffCommand : Outport
  landCommand : Outport  Port=2
  wires:
  Rate Transition3/1 -> NOT/1  "takeoff"
  Clock/1 -> Compare To Constant/1
  Compare To Constant/1 -> Rate Transition3/1
  Compare To Constant1/1 -> Rate Transition1/1
  Clock1/1 -> Compare To Constant1/1
  Rate Transition1/1 -> NOT1/1  "land"
  NOT/1 -> takeoffCommand/1
  NOT1/1 -> landCommand/1

== matlab function flightControlSystem/Flight Control System/Position//Attitude Reference Input/ /keyboard Commands/MATLAB Function ==
  data: keyboardRead input; landCommand output; takeoffCommand output; enableLanding input
function [landCommand, takeoffCommand] = keyboardRead(keyboardRead,enableLanding)

keyboardReadStr=char(keyboardRead);

landCommand = enableLanding &&( (keyboardReadStr == "l") || (keyboardReadStr == "L") );

takeoffCommand = (keyboardReadStr == "s") || (keyboardReadStr == "S");

== matlab function flightControlSystem/Flight Control System/landing logic/MATLAB Function1 ==
  data: x output; y output; landCommand input; posRef input; altitudeRef output; Ts input; landingAltitude input
function [x, y, altitudeRef] =land(landCommand, posRef, Ts, landingAltitude)
%landCommand is either 1(true) or 0(false)

%posRef is the target position (where we want to go) [x,y,z] vector

%Ts is the sampling period for how often the drone its own position using
%its onboard sensors

%landingAltitude is the target z coordinate when landCommand = true


% altitudeRef=posRef(3);
% 
% if landCommand
%     
%     % altitude is negative!
% %     altitudeRef = altitudeRef + Ts*0.1;
%     
%     % altitudeRef=landingAltitude;
%     altitudeRef=single(0);
%     
%     
%     if altitudeRef>=0  % if landed on the ground then stay
%         altitudeRef=single(0);
%     end
% end
% 
% posRef(3)=altitudeRef;

if landCommand
    altitudeRef = landingAltitude;
    
else
    altitudeRef = posRef(3); % z coordinate of position reference
end
x = posRef(1);
y = posRef(2);
end

== matlab function flightControlSystem/Flight Control System/Crash Predictor Flags/MATLAB Function1 ==
  data: dx input; dy input; Y input; opticalFlow_data input; estimatorPosVisDeltaXYMax input; crashFlagOut output; takeoffCommand input
function crashFlagOut  = crashPredictor(dx, dy, Y, opticalFlow_data, estimatorPosVisDeltaXYMax, takeoffCommand)


if ~takeoffCommand
    % if takeoff is not started (takeoffCommand not given) crashFlag should be 0
    
    crashFlag=0;
    
else
    % Geofencing error
    geofencingError= abs(dx)>10 || abs(Y)>10;
    
    
    if geofencingError % Geofencing error
        crashFlag = 1;
        
    else
        
        % estimator/Optical flow error
        estimatorOrOpticaFlowError =  ...
            ( (abs(estimatorPosVisDeltaXYMax) > 0.01) ...
            && (abs (opticalFlow_data(1) * estimatorPosVisDeltaXYMax - dx ) > 6)   ) ...
            || ...
            ( (abs ( opticalFlow_data(2) * estimatorPosVisDeltaXYMax - dy ) > 6) ...
            && (abs ( opticalFlow_data(2) ) > 0.01) );
        
        if estimatorOrOpticaFlowError % estimator/Optical flow error
            
            crashFlag = 99;
            
        else % Normal condition
            crashFlag=0;
        end
        
        
        
    end
end
crashFlagOut=uint8(crashFlag); % because output is uint8

end
